simulink library "lib_dGrid"  (R2023b)
settings: Solver=VariableStepAuto  StartTime=0.0  StopTime=10.0  RelTol=1e-3
values from neighbouring files (symbols this model uses):
  C_PM = 10e-3    (= 0.01)    [my_MMC_param.m]
  Cbase = 1/Zbase/wb    (= 3.10849498226e-05)    [my_MMC_param.m]
  f0 = 50/fb    (= 1)    [my_MMC_param.m]
  Fn_filter = 1000    [my_MMC_param.m]
  Fnom = 50    [my_MMC_param.m]
  GFL_APC = 1    [Analysis_Main.m]    (also in initSimu.m; my_MMC_param.m)
  GFL_DVC = 2    [Analysis_Main.m]    (also in initSimu.m; my_MMC_param.m)
  GFM_APC = 3; (values programmed in EMT models)    [Analysis_Main.m]    (also in initSimu.m; my_MMC_param.m = 3)
  GFM_VF = 0    [my_MMC_param.m]
  Ibase = 2*Sbase/(3*Ubase)    [my_MMC_param.m]
  Idcb = Sbase/Udcb    [my_MMC_param.m]
  Ki_Iccsc = 5.15    [my_MMC_param.m]
  Ki_Ireg = CCCTRL.CC.ki    [my_MMC_param.m]
  Ki_Izscc = 100    [my_MMC_param.m]
  Ki_PLL = 1/(CCCTRL.PLL.v0*CCCTRL.PLL.T^2)    [my_MMC_param.m]
  Ki_Preg = 1.0*10    (= 10)    [my_MMC_param.m]
  Ki_Qreg = 1.0*10    (= 10)    [my_MMC_param.m]
  Ki_VAC_GFL = 50    [my_MMC_param.m]
  Ki_VACreg = 10    [my_MMC_param.m]
  Ki_VDCreg = 10    [my_MMC_param.m]
  Ki_WtReg = Kp_WtReg / 0.025    (= 1600)    [my_MMC_param.m]
  Kp_Iccsc = 0.21    [my_MMC_param.m]
  Kp_Ireg = CCCTRL.CC.kp    [my_MMC_param.m]
  Kp_Izscc = 10    [my_MMC_param.m]
  Kp_PLL = 2/CCCTRL.PLL.v0/CCCTRL.PLL.T    [my_MMC_param.m]
  Kp_Preg = 0.5/3*1    (= 0.166666666667)    [my_MMC_param.m]
  Kp_Qreg = 0.5/3*1    (= 0.166666666667)    [my_MMC_param.m]
  Kp_VAC_GFL = 0.5    [my_MMC_param.m]
  Kp_VACreg = 0.01    [my_MMC_param.m]
  Kp_VDCreg = 1    [my_MMC_param.m]
  Kp_WtReg = 40    [my_MMC_param.m]
  Kpv_GFM = 1    [my_MMC_param.m]
  Kpwm = 0.5    [my_MMC_param.m]
  Larm = Larm_pu*(Zbase/wb)    (= 0.0488923985178)    [my_MMC_param.m]
  Lff = Larm_pu/2    (= 0.075)    [my_MMC_param.m]
  Limits_Ireg = [ 2.0  -2.0]    [my_MMC_param.m]
  Limits_Preg = [ 2, -2 ]    [my_MMC_param.m]
  Limits_Qreg = 2*[ 0.42, -0.42 ]    [my_MMC_param.m]
  Limits_VACreg = [ 1.3  -1.3]    [my_MMC_param.m]
  Limits_VDCreg = [ 2.0  -2.0]    [my_MMC_param.m]
  MMC1 = MMC    [Analysis_Main.m]    (also in initSimu.m)
  Nb_PM = 400    [my_MMC_param.m]
  PhaseDelay = 1.0*Ts_Control*2*pi*50    (= 0.0628318530718)    [my_MMC_param.m]
  Pnom = 1000e6    (= 1000000000)    [my_MMC_param.m]
  Rarm = Rarm_pu*Zbase    (= 0.1536)    [my_MMC_param.m]
  Slope_Pref = 0.5    [my_MMC_param.m]
  Slope_Qref = 0.5    [my_MMC_param.m]
  Slope_Vdc_ref = Vnom_dc/2    (= 320000)    [my_MMC_param.m]
  Tdeblock = 1.5    [my_MMC_param.m]
  Ton_CROSSreg = Ton_PQreg+3    (= 7)    [my_MMC_param.m]
  Ton_PQreg = 4    [my_MMC_param.m]
  Ton_VDCreg = 1.5    [my_MMC_param.m]
  Ts = Ts_Control    (= 0.0002)    [my_MMC_param.m]
  Ts_Control = Ts_Power*2    (= 0.0002)    [my_MMC_param.m]
  Ts_Power = 20e-6 * 5    (= 0.0001)    [my_MMC_param.m]
  Ubase = sqrt(2/3)*Vnom_sec    [my_MMC_param.m]
  Udcb = 2*Ubase    [my_MMC_param.m]
  Vc0_PM = 0    [my_MMC_param.m]
  Vnom_dc = 640e3    (= 640000)    [my_MMC_param.m]
  Vnom_sec = 320e3    (= 320000)    [my_MMC_param.m]
  wb = 2*pi*fb    (= 314.159265359)    [my_MMC_param.m]
  Wt_ref_pu = 0.5 * C_PM * (Vnom_dc/Nb_PM)^2 * Nb_PM * 6 / Pnom    (= 0.03072)    [my_MMC_param.m]
undefined symbols (not defined in the file or in its folder): ControlSampleTime, DiscIntNeverNeededParam, MMC, PLL, VSM
libraries: simulink x50, spsCurrentMeasurementLib x20, spsSecondOrderFilterLib x20, spsDiodeLib x12, spsControlledVoltageSourceLib x12, spsSeriesRLCBranchLib x10, spsFirstOrderFilterLib x9, spsVoltageMeasurementLib x8, spsMeanLib x7, FriedrichLibrary x6, $bdroot x6, powerlib_extras x4
(part 2 of 8)

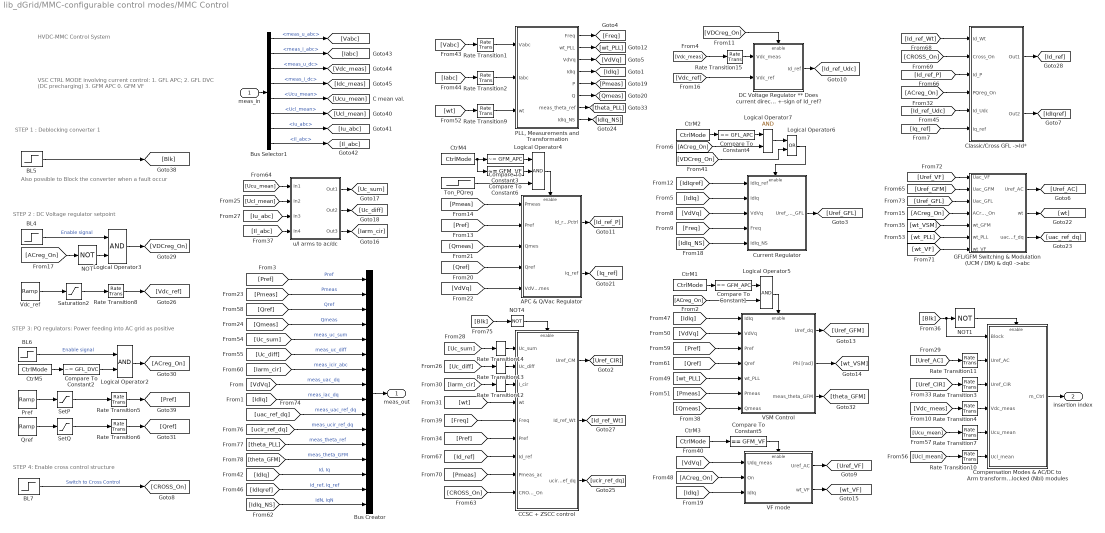
== system lib_dGrid/MMC-configurable control modes/MMC Control ==
  note: HVDC-MMC Control System
  note: VSC CTRL MODE involving current control:
      | 1. GFL APC; 2. GFL DVC  (DC precharging)
      | 3. GFM APC
      | 0. GFM VF
  note: STEP 4: Enable cross control structure
  note: STEP 2 : DC Voltage regulator setpoint
  note: Also possible to Block the converter when a fault occur
  note: STEP 1 : Deblocking converter 1
  note: STEP 3: PQ regulators: Power feeding into
      | AC grid as positive
  meas_in : Inport
  APC & Q/Vac Regulator : Subsystem
  BL4 : Step  Time=Ton_VDCreg  SampleTime=Ts
  BL5 : Step  Time=Tdeblock  Before=1  After=0  SampleTime=Ts_Power
  BL6 : Step  Time=Ton_PQreg  SampleTime=Ts
  BL7 : Step  Time=Ton_CROSSreg  SampleTime=Ts
  Bus Creator : BusCreator  Inputs=16
  Bus Selector1 : BusSelector  OutputSignals=meas_u_abc,meas_i_abc,meas_u_dc,meas_i_dc,Ucu_mean,Ucl_mean,Iu_abc,Il_abc
  CCSC + ZSCC control : Subsystem
  Classic/Cross GFL ->Id* : Subsystem
  Compare To Constant1 : simulink/Logic and Bit Operations/Compare To Constant  relop===  const=GFM_APC  OutDataTypeStr=boolean
  Compare To Constant2 : simulink/Logic and Bit Operations/Compare To Constant  relop=~=  const=GFL_DVC  OutDataTypeStr=boolean
  Compare To Constant3 : simulink/Logic and Bit Operations/Compare To Constant  relop=~=  const=GFM_APC  OutDataTypeStr=boolean
  Compare To Constant4 : simulink/Logic and Bit Operations/Compare To Constant  relop===  const=GFL_APC  OutDataTypeStr=boolean
  Compare To Constant5 : simulink/Logic and Bit Operations/Compare To Constant  relop===  const=GFM_VF  OutDataTypeStr=boolean
  Compare To Constant6 : simulink/Logic and Bit Operations/Compare To Constant  relop=~=  const=GFM_VF  OutDataTypeStr=boolean
  Compensation Modes & AC/DC to Arm transform Number of inserted (Nin) and blocked (Nbl) modules : Subsystem
  CtrM{1..5} (5 alike) : Constant  Value=CtrlMode
  Current Regulator : Subsystem
  DC Voltage Regulator ** Does current direction influence the +-sign of Id_ref? : Subsystem
  GFL/GFM Switching & Modulation (UCM / DM) & dq0 ->abc : Subsystem
  Logical Operator{2..3,5,7} (4 alike) : Logic  AllPortsSameDT=off  OutDataTypeStr=float('double')
  Logical Operator4 : Logic  Inputs=3  AllPortsSameDT=off  OutDataTypeStr=float('double')
  Logical Operator6 : Logic  Operator=OR  AllPortsSameDT=off  OutDataTypeStr=float('double')
  NOT : Logic  Operator=NOT  IconShape=distinctive  AllPortsSameDT=off  OutDataTypeStr=boolean
  NOT1 : Logic  Operator=NOT  IconShape=distinctive  AllPortsSameDT=off  OutDataTypeStr=boolean
  NOT4 : Logic  Operator=NOT  IconShape=distinctive  AllPortsSameDT=off  OutDataTypeStr=boolean
  "PLL, Measurements and Transformation" : Subsystem
  Pref : simulink/Sources/Ramp  slope=Slope_Pref * sign(Set.Pref)  start=Tramping_Pref  InitialOutput=0
  Qref : simulink/Sources/Ramp  slope=Slope_Qref  start=Tramping_Qref  InitialOutput=0
  Rate Transition{1..2,5..6,8..9,12..15} (10 alike) : RateTransition  OutPortSampleTime=Ts_Control
  Rate Transition{3..4,7,10..11} (5 alike) : RateTransition  Deterministic=off  OutPortSampleTime=Ts_Power
  Saturation2 : Saturate  UpperLimit=Vnom_dc  LowerLimit=eps
  SetP : Saturate  UpperLimit=abs(Set.Pref)  LowerLimit=-abs(Set.Pref)
  SetQ : Saturate  UpperLimit=Set.Qref  LowerLimit=-Set.Qref
  Ton_PQreg : Step  Time=Ton_PQreg  SampleTime=Ts
  VF mode : Subsystem
  VSM Control : Subsystem
  "Vdc_ref " : simulink/Sources/Ramp  slope=Slope_Vdc_ref  start=Tramping_Vdc_ref  InitialOutput=Vnom_sec*1.37
  u/l arms to ac/dc : Subsystem
  meas_out : Outport  VectorParamsAs1DForOutWhenUnconnected=off
  insertion index : Outport  Port=2  VectorParamsAs1DForOutWhenUnconnected=off
  wires:
  [Vabc] -> Rate Transition1/1
  [Iabc] -> Rate Transition2/1
  DC Voltage Regulator ** Does current direction influence the +-sign of Id_ref?/1(Id_ref) -> [Id_ref_Udc]
  "PLL, Measurements and Transformation"/2(wt_PLL) -> [wt_PLL]
  "PLL, Measurements and Transformation"/4(IdIq) -> [IdIq]
  [Freq] -> Current Regulator/4(Freq)
  "PLL, Measurements and Transformation"/3(VdVq) -> [VdVq]
  [IdIq] -> Current Regulator/2(IdIq)
  "PLL, Measurements and Transformation"/1(Freq) -> [Freq]
  [VdVq] -> Current Regulator/3(VdVq)
  Rate Transition2/1 -> "PLL, Measurements and Transformation"/2(Iabc)
  Rate Transition1/1 -> "PLL, Measurements and Transformation"/1(Vabc)
  [Vdc_ref] -> DC Voltage Regulator ** Does current direction influence the +-sign of Id_ref?/2(Vdc_ref)
  [VDCreg_On] -> DC Voltage Regulator ** Does current direction influence the +-sign of Id_ref?/Enable
  "PLL, Measurements and Transformation"/5(P) -> [Pmeas]
  [VdVq] -> APC & Q/Vac Regulator/5(VdVq_mes)
  [Qmeas] -> APC & Q/Vac Regulator/3(Qmes)
  "PLL, Measurements and Transformation"/6(Q) -> [Qmeas]
  [Qref] -> APC & Q/Vac Regulator/4(Qref)
  [Uc_diff] -> Rate Transition13/1
  [Iarm_cir] -> Rate Transition12/1
  [Uc_sum] -> Rate Transition14/1
  [Uref_CIR] -> Rate Transition3/1
  Rate Transition11/1 -> Compensation Modes & AC/DC to Arm transform Number of inserted (Nin) and blocked (Nbl) modules/2(Uref_AC)
  Rate Transition3/1 -> Compensation Modes & AC/DC to Arm transform Number of inserted (Nin) and blocked (Nbl) modules/3(Uref_CIR)
  APC & Q/Vac Regulator/1(Id_ref_Pctrl) -> [Id_ref_P]
  [VdVq] -> VSM Control/2(VdVq)
  VSM Control/1(Uref_dq) -> [Uref_GFM]
  [IdIq] -> VSM Control/1(IdIq)
  [Pref] -> VSM Control/3(Pref)
  [wt_PLL] -> VSM Control/5(wt_PLL)
  [wt] -> Rate Transition9/1
  [Freq] -> CCSC + ZSCC control/5(Freq)
  [Pref] -> CCSC + ZSCC control/6(Pref)
  [Vdc_meas] -> Rate Transition4/1
  Rate Transition4/1 -> Compensation Modes & AC/DC to Arm transform Number of inserted (Nin) and blocked (Nbl) modules/4(Vdc_meas)
  CCSC + ZSCC control/2(Id_ref_Wt) -> [Id_ref_Wt]
  [Id_ref] -> CCSC + ZSCC control/7(Id_ref)
  [Pmeas] -> CCSC + ZSCC control/8(Pmeas_ac)
  Rate Transition9/1 -> "PLL, Measurements and Transformation"/3(wt)
  VSM Control/2(Phi [rad]) -> [wt_VSM]
  [wt] -> CCSC + ZSCC control/4(wt)
  [Pmeas] -> VSM Control/6(Pmeas)
  [Qmeas] -> VSM Control/7(Qmeas)
  [Uc_diff] -> Bus Creator/6  "meas_uc_diff"
  [Uc_sum] -> Bus Creator/5  "meas_uc_sum"
  [Iarm_cir] -> Bus Creator/7  "meas_icir_abc"
  Bus Creator/1 -> meas_out/1
  Rate Transition6/1 -> [Qref]
  BL6/1 -> Logical Operator2/1  "Enable signal"
  Pref/1 -> SetP/1
  SetP/1 -> Rate Transition5/1
  BL5/1 -> [Blk]
  BL4/1 -> Logical Operator3/1  "Enable signal"
  Saturation2/1 -> Rate Transition8/1
  BL7/1 -> [CROSS_On]  "Switch to Cross Control"
  "Vdc_ref "/1 -> Saturation2/1
  Rate Transition8/1 -> [Vdc_ref]
  SetQ/1 -> Rate Transition6/1
  Rate Transition5/1 -> [Pref]
  Qref/1 -> SetQ/1
  [CROSS_On] -> CCSC + ZSCC control/9(CROSS_On)
  meas_in/1 -> Bus Selector1/1
  Bus Selector1/7 -> [Iu_abc]  "<Iu_abc>"
  Bus Selector1/8 -> [Il_abc]  "<Il_abc>"
  Bus Selector1/6 -> [Ucl_mean]  "<Ucl_mean>"
  Bus Selector1/5 -> [Ucu_mean]  "<Ucu_mean>"
  Bus Selector1/1 -> [Vabc]  "<meas_u_abc>"
  Bus Selector1/2 -> [Iabc]  "<meas_i_abc>"
  Bus Selector1/3 -> [Vdc_meas]  "<meas_u_dc>"
  Bus Selector1/4 -> [Idc_meas]  "<meas_i_dc>"
  Compensation Modes & AC/DC to Arm transform Number of inserted (Nin) and blocked (Nbl) modules/1(m_Ctrl) -> insertion index/1
  [Ucu_mean] -> Rate Transition7/1
  [Ucl_mean] -> Rate Transition10/1
  Rate Transition7/1 -> Compensation Modes & AC/DC to Arm transform Number of inserted (Nin) and blocked (Nbl) modules/5(Ucu_mean)
  Rate Transition10/1 -> Compensation Modes & AC/DC to Arm transform Number of inserted (Nin) and blocked (Nbl) modules/6(Ucl_mean)
  CCSC + ZSCC control/1(Uref_CM) -> [Uref_CIR]
  [Blk] -> Compensation Modes & AC/DC to Arm transform Number of inserted (Nin) and blocked (Nbl) modules/1(Block), NOT1/1
  [Pref] -> Bus Creator/1  "Pref"
  [Pmeas] -> Bus Creator/2  "Pmeas"
  [Qref] -> Bus Creator/3  "Qref"
  [Qmeas] -> Bus Creator/4  "Qmeas"
  [Pmeas] -> APC & Q/Vac Regulator/1(Pmeas)
  [Pref] -> APC & Q/Vac Regulator/2(Pref)
  APC & Q/Vac Regulator/2(Iq_ref) -> [Iq_ref]
  Compare To Constant2/1 -> Logical Operator2/2
  Logical Operator2/1 -> [ACreg_On]
  [IdIqref] -> Current Regulator/1(IdIq_ref)
  [Id_ref_Wt] -> Classic/Cross GFL ->Id*/1(Id_Wt)
  [CROSS_On] -> Classic/Cross GFL ->Id*/2(Cross_On)
  [Id_ref_P] -> Classic/Cross GFL ->Id*/3(Id_P)
  [ACreg_On] -> Classic/Cross GFL ->Id*/4(PQreg_On)
  [Id_ref_Udc] -> Classic/Cross GFL ->Id*/5(Id_Udc)
  [Iq_ref] -> Classic/Cross GFL ->Id*/6(Iq_ref)
  Classic/Cross GFL ->Id*/1(Out1) -> [Id_ref]
  Classic/Cross GFL ->Id*/2(Out2) -> [IdIqref]
  Logical Operator3/1 -> [VDCreg_On]
  NOT/1 -> Logical Operator3/2
  [ACreg_On] -> NOT/1
  NOT1/1 -> Compensation Modes & AC/DC to Arm transform Number of inserted (Nin) and blocked (Nbl) modules/Enable
  [ACreg_On] -> Logical Operator5/2
  CtrM1/1 -> Compare To Constant1/1
  Compare To Constant1/1 -> Logical Operator5/1
  Logical Operator5/1 -> VSM Control/Enable
  [Qref] -> VSM Control/4(Qref)
  [Uref_AC] -> Rate Transition11/1
  [Uref_GFM] -> GFL/GFM Switching & Modulation (UCM / DM) & dq0 ->abc/2(Uac_GFM)
  [Uref_GFL] -> GFL/GFM Switching & Modulation (UCM / DM) & dq0 ->abc/3(Uac_GFL)
  [ACreg_On] -> GFL/GFM Switching & Modulation (UCM / DM) & dq0 ->abc/4(ACreg_On)
  [wt_VSM] -> GFL/GFM Switching & Modulation (UCM / DM) & dq0 ->abc/5(wt_GFM)
  [wt_PLL] -> GFL/GFM Switching & Modulation (UCM / DM) & dq0 ->abc/6(wt_PLL)
  GFL/GFM Switching & Modulation (UCM / DM) & dq0 ->abc/1(Uref_AC) -> [Uref_AC]
  GFL/GFM Switching & Modulation (UCM / DM) & dq0 ->abc/2(wt) -> [wt]
  [Ucu_mean] -> u/l arms to ac/dc/1(In1)
  [Ucl_mean] -> u/l arms to ac/dc/2(In2)
  [Iu_abc] -> u/l arms to ac/dc/3(In3)
  [Il_abc] -> u/l arms to ac/dc/4(In4)
  u/l arms to ac/dc/1(Out1) -> [Uc_sum]
  u/l arms to ac/dc/2(Out2) -> [Uc_diff]
  u/l arms to ac/dc/3(Out3) -> [Iarm_cir]
  [wt_VF] -> GFL/GFM Switching & Modulation (UCM / DM) & dq0 ->abc/7(wt_VF)
  [Uref_VF] -> GFL/GFM Switching & Modulation (UCM / DM) & dq0 ->abc/1(Uac_VF)
  CCSC + ZSCC control/3(ucir_ref_dq) -> [ucir_ref_dq]
  [ucir_ref_dq] -> Bus Creator/11  "meas_ucir_ref_dq"
  [VdVq] -> Bus Creator/8  "meas_uac_dq"
  [IdIq] -> Bus Creator/9  "meas_iac_dq"
  [uac_ref_dq] -> Bus Creator/10  "meas_uac_ref_dq"
  [theta_PLL] -> Bus Creator/12  "meas_theta_ref"
  [theta_GFM] -> Bus Creator/13  "meas_theta_GFM"
  VSM Control/3(meas_theta_GFM) -> [theta_GFM]
  "PLL, Measurements and Transformation"/7(meas_theta_ref) -> [theta_PLL]
  Current Regulator/1(Uref_AC_GFL) -> [Uref_GFL]
  GFL/GFM Switching & Modulation (UCM / DM) & dq0 ->abc/3(uac_ref_dq) -> [uac_ref_dq]
  [ACreg_On] -> Logical Operator7/2
  [VDCreg_On] -> Logical Operator6/2
  Logical Operator6/1 -> Current Regulator/Enable
  CtrM3/1 -> Compare To Constant5/1
  Compare To Constant5/1 -> VF mode/Enable
  [ACreg_On] -> VF mode/2(On)
  VF mode/2(wt_VF) -> [wt_VF]
  VF mode/1(Uref_AC) -> [Uref_VF]
  [VdVq] -> VF mode/1(Udq_meas)
  [Blk] -> NOT4/1
  NOT4/1 -> CCSC + ZSCC control/Enable
  Ton_PQreg/1 -> Logical Operator4/3
  CtrM2/1 -> Compare To Constant4/1
  Compare To Constant4/1 -> Logical Operator7/1
  Logical Operator7/1 -> Logical Operator6/1
  [IdIq] -> Bus Creator/14  "Id, Iq"
  [IdIqref] -> Bus Creator/15  "Id_ref, Iq_ref"
  Rate Transition12/1 -> CCSC + ZSCC control/3(I_cir)
  Rate Transition13/1 -> CCSC + ZSCC control/2(Uc_diff)
  Rate Transition14/1 -> CCSC + ZSCC control/1(Uc_sum)
  Rate Transition15/1 -> DC Voltage Regulator ** Does current direction influence the +-sign of Id_ref?/1(Vdc_meas)
  [Vdc_meas] -> Rate Transition15/1
  [IdIq] -> VF mode/3(IdIq)
  CtrM5/1 -> Compare To Constant2/1
  CtrM4/1 -> Compare To Constant6/1, Compare To Constant3/1
  Compare To Constant3/1 -> Logical Operator4/1
  Compare To Constant6/1 -> Logical Operator4/2
  Logical Operator4/1 -> APC & Q/Vac Regulator/Enable
  "PLL, Measurements and Transformation"/8(IdIq_NS) -> [IdIq_NS]
  [IdIq_NS] -> Bus Creator/16  "IdN, IqN"
  [IdIq_NS] -> Current Regulator/5(IdIq_NS)

== system lib_dGrid/MMC-configurable control modes/Subsystem ==
  Current Measurement1 : spsCurrentMeasurementLib/Current Measurement  PhasorSimulation=off  OutputType=Complex  PSBequivalent=0
  Goto19 : Goto  Commented=on  GotoTag=V12_Ap
  Voltage Measurement : spsVoltageMeasurementLib/Voltage Measurement  Commented=on  PhasorSimulation=off  OutputType=Complex  PSBequivalent=0
  I1 : PMIOPort  Side=Left
  I2 : PMIOPort  Port=2  Side=Left
  O1 : PMIOPort  Port=3  Side=Right
  O2 : PMIOPort  Port=4  Side=Right
  I_Ap : Outport  VectorParamsAs1DForOutWhenUnconnected=off
  wires:
  Current Measurement1/1 -> I_Ap/1
  Voltage Measurement/1 -> Goto19/1
  connections:
  Current Measurement1/RConn1 -- Voltage Measurement/LConn1 -- I1/RConn1
  Current Measurement1/LConn1 -- O1/RConn1
  I2/RConn1 -- Voltage Measurement/LConn2 -- O2/RConn1

== system lib_dGrid/MMC-configurable control modes/Subsystem1 ==
  Current Measurement1 : spsCurrentMeasurementLib/Current Measurement  PhasorSimulation=off  OutputType=Complex  PSBequivalent=0
  Goto19 : Goto  Commented=on  GotoTag=V12_Am
  Voltage Measurement : spsVoltageMeasurementLib/Voltage Measurement  Commented=on  PhasorSimulation=off  OutputType=Complex  PSBequivalent=0
  I1 : PMIOPort  Side=Left
  I2 : PMIOPort  Port=2  Side=Left
  O1 : PMIOPort  Port=3  Side=Right
  O2 : PMIOPort  Port=4  Side=Right
  I_Am : Outport  VectorParamsAs1DForOutWhenUnconnected=off
  wires:
  Voltage Measurement/1 -> Goto19/1
  Current Measurement1/1 -> I_Am/1
  connections:
  Voltage Measurement/LConn2 -- O2/RConn1 -- I2/RConn1
  Current Measurement1/LConn1 -- O1/RConn1
  Voltage Measurement/LConn1 -- Current Measurement1/RConn1 -- I1/RConn1

== system lib_dGrid/MMC-configurable control modes/Subsystem2 ==
  Current Measurement1 : spsCurrentMeasurementLib/Current Measurement  PhasorSimulation=off  OutputType=Complex  PSBequivalent=0
  Goto19 : Goto  Commented=on  GotoTag=V12_Bp
  Voltage Measurement : spsVoltageMeasurementLib/Voltage Measurement  Commented=on  PhasorSimulation=off  OutputType=Complex  PSBequivalent=0
  I1 : PMIOPort  Side=Left
  I2 : PMIOPort  Port=2  Side=Left
  O1 : PMIOPort  Port=3  Side=Right
  O2 : PMIOPort  Port=4  Side=Right
  I_Bp : Outport  VectorParamsAs1DForOutWhenUnconnected=off
  wires:
  Voltage Measurement/1 -> Goto19/1
  Current Measurement1/1 -> I_Bp/1
  connections:
  Voltage Measurement/LConn2 -- O2/RConn1 -- I2/RConn1
  Current Measurement1/LConn1 -- O1/RConn1
  Voltage Measurement/LConn1 -- Current Measurement1/RConn1 -- I1/RConn1

== system lib_dGrid/MMC-configurable control modes/Subsystem3 ==
  Current Measurement1 : spsCurrentMeasurementLib/Current Measurement  PhasorSimulation=off  OutputType=Complex  PSBequivalent=0
  Goto19 : Goto  Commented=on  GotoTag=V12_Bm
  Voltage Measurement : spsVoltageMeasurementLib/Voltage Measurement  Commented=on  PhasorSimulation=off  OutputType=Complex  PSBequivalent=0
  I1 : PMIOPort  Side=Left
  I2 : PMIOPort  Port=2  Side=Left
  O1 : PMIOPort  Port=3  Side=Right
  O2 : PMIOPort  Port=4  Side=Right
  I_Bm : Outport  VectorParamsAs1DForOutWhenUnconnected=off
  wires:
  Current Measurement1/1 -> I_Bm/1
  Voltage Measurement/1 -> Goto19/1
  connections:
  I1/RConn1 -- Current Measurement1/RConn1 -- Voltage Measurement/LConn1
  Current Measurement1/LConn1 -- O1/RConn1
  I2/RConn1 -- O2/RConn1 -- Voltage Measurement/LConn2

== system lib_dGrid/MMC-configurable control modes/Subsystem4 ==
  Current Measurement1 : spsCurrentMeasurementLib/Current Measurement  PhasorSimulation=off  OutputType=Complex  PSBequivalent=0
  Goto19 : Goto  Commented=on  GotoTag=V12_Cp
  Voltage Measurement : spsVoltageMeasurementLib/Voltage Measurement  Commented=on  PhasorSimulation=off  OutputType=Complex  PSBequivalent=0
  I1 : PMIOPort  Side=Left
  I2 : PMIOPort  Port=2  Side=Left
  O1 : PMIOPort  Port=3  Side=Right
  O2 : PMIOPort  Port=4  Side=Right
  I_Cp : Outport  VectorParamsAs1DForOutWhenUnconnected=off
  wires:
  Current Measurement1/1 -> I_Cp/1
  Voltage Measurement/1 -> Goto19/1
  connections:
  I1/RConn1 -- Current Measurement1/RConn1 -- Voltage Measurement/LConn1
  Current Measurement1/LConn1 -- O1/RConn1
  I2/RConn1 -- O2/RConn1 -- Voltage Measurement/LConn2

== system lib_dGrid/MMC-configurable control modes/Subsystem5 ==
  Current Measurement1 : spsCurrentMeasurementLib/Current Measurement  PhasorSimulation=off  OutputType=Complex  PSBequivalent=0
  Goto19 : Goto  Commented=on  GotoTag=V12_Cm
  Voltage Measurement : spsVoltageMeasurementLib/Voltage Measurement  Commented=on  PhasorSimulation=off  OutputType=Complex  PSBequivalent=0
  I1 : PMIOPort  Side=Left
  I2 : PMIOPort  Port=2  Side=Left
  O1 : PMIOPort  Port=3  Side=Right
  O2 : PMIOPort  Port=4  Side=Right
  I_Cm : Outport  VectorParamsAs1DForOutWhenUnconnected=off
  wires:
  Voltage Measurement/1 -> Goto19/1
  Current Measurement1/1 -> I_Cm/1
  connections:
  Voltage Measurement/LConn2 -- O2/RConn1 -- I2/RConn1
  Current Measurement1/LConn1 -- O1/RConn1
  Voltage Measurement/LConn1 -- Current Measurement1/RConn1 -- I1/RConn1

== system lib_dGrid/TL-VSC-configurable control modes/Filters 60Hz2 ==
  note: High-pass
      | damped filters
  note: AC Filters, 40 Mvar @ 100 kV
  "27th 18 Mvar Q = 15 " : spsThreePhaseHarmonicFilterLib/Three-Phase Harmonic Filter  LConnTagsString=A|B|C  FilterType=High-pass  FilterConnection=Y (grounded)  ParNom="[320e3  Fnom]"  Qc=0.2*Pnom * 0.45  Fr=27*Fnom  Frd=[11*60 13*60]  Q=15  Measurements=None
      settings: AttributesFormatString=\n
  "54th 22 Mvar Q = 15 " : spsThreePhaseHarmonicFilterLib/Three-Phase Harmonic Filter  LConnTagsString=A|B|C  FilterType=High-pass  FilterConnection=Y (grounded)  ParNom="[320e3  Fnom]"  Qc=0.2*Pnom * 0.55  Fr=(2*27)*Fnom  Frd=[11*60 13*60]  Q=15  Measurements=None
      settings: AttributesFormatString=\n
  A : PMIOPort  Side=Left
  B : PMIOPort  Port=2  Side=Left
  C : PMIOPort  Port=3  Side=Left
  connections:
  "54th 22 Mvar Q = 15 "/LConn3 -- C/RConn1 -- "27th 18 Mvar Q = 15 "/LConn3
  "54th 22 Mvar Q = 15 "/LConn2 -- B/RConn1 -- "27th 18 Mvar Q = 15 "/LConn2
  "54th 22 Mvar Q = 15 "/LConn1 -- A/RConn1 -- "27th 18 Mvar Q = 15 "/LConn1

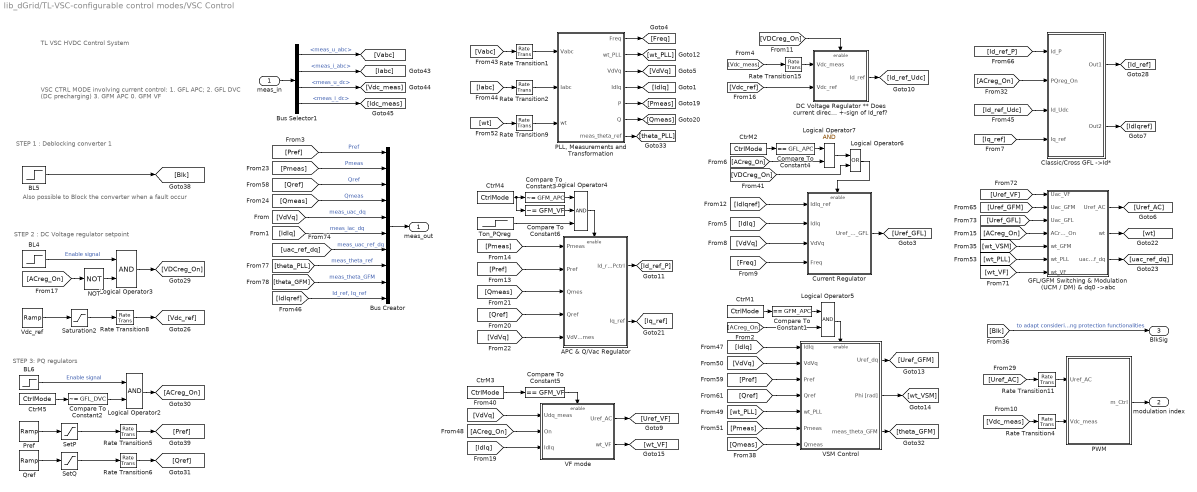
== system lib_dGrid/TL-VSC-configurable control modes/VSC Control ==
  note: TL VSC HVDC
      | Control System
  note: VSC CTRL MODE involving current control:
      | 1. GFL APC; 2. GFL DVC  (DC precharging)
      | 3. GFM APC
      | 0. GFM VF
  note: STEP 2 : DC Voltage regulator setpoint
  note: Also possible to Block the converter when a fault occur
  note: STEP 1 : Deblocking converter 1
  note: STEP 3: PQ regulators
  meas_in : Inport
  APC & Q/Vac Regulator : Subsystem
  BL4 : Step  Time=Ton_VDCreg  SampleTime=Ts
  BL5 : Step  Time=Tdeblock  Before=1  After=0  SampleTime=Ts_Power
  BL6 : Step  Time=Ton_PQreg  SampleTime=Ts
  Bus Creator : BusCreator  Inputs=10
  Bus Selector1 : BusSelector  OutputSignals=meas_u_abc,meas_i_abc,meas_u_dc,meas_i_dc
  Classic/Cross GFL ->Id* : Subsystem
  Compare To Constant1 : simulink/Logic and Bit Operations/Compare To Constant  relop===  const=GFM_APC  OutDataTypeStr=boolean
  Compare To Constant2 : simulink/Logic and Bit Operations/Compare To Constant  relop=~=  const=GFL_DVC  OutDataTypeStr=boolean
  Compare To Constant3 : simulink/Logic and Bit Operations/Compare To Constant  relop=~=  const=GFM_APC  OutDataTypeStr=boolean
  Compare To Constant4 : simulink/Logic and Bit Operations/Compare To Constant  relop===  const=GFL_APC  OutDataTypeStr=boolean
  Compare To Constant5 : simulink/Logic and Bit Operations/Compare To Constant  relop===  const=GFM_VF  OutDataTypeStr=boolean
  Compare To Constant6 : simulink/Logic and Bit Operations/Compare To Constant  relop=~=  const=GFM_VF  OutDataTypeStr=boolean
  CtrM{1..5} (5 alike) : Constant  Value=CtrlMode
  Current Regulator : Subsystem
  DC Voltage Regulator ** Does current direction influence the +-sign of Id_ref? : Subsystem
  GFL/GFM Switching & Modulation (UCM / DM) & dq0 ->abc : Subsystem
  Logical Operator{2..3,5,7} (4 alike) : Logic  AllPortsSameDT=off  OutDataTypeStr=float('double')
  Logical Operator4 : Logic  Inputs=3  AllPortsSameDT=off  OutDataTypeStr=float('double')
  Logical Operator6 : Logic  Operator=OR  AllPortsSameDT=off  OutDataTypeStr=float('double')
  NOT : Logic  Operator=NOT  IconShape=distinctive  AllPortsSameDT=off  OutDataTypeStr=boolean
  "PLL, Measurements and Transformation" : Subsystem
  PWM : Subsystem
  Pref : simulink/Sources/Ramp  slope=Slope_Pref  start=Tramping_Pref  InitialOutput=0
  Qref : simulink/Sources/Ramp  slope=Slope_Qref  start=Tramping_Qref  InitialOutput=0
  Rate Transition{1..2,5..6,8..9,15} (7 alike) : RateTransition  OutPortSampleTime=Ts_Control
  Rate Transition11 : RateTransition  Deterministic=off  OutPortSampleTime=Ts_Power
  Rate Transition4 : RateTransition  Deterministic=off  OutPortSampleTime=Ts_Power
  Saturation2 : Saturate  UpperLimit=Vnom_dc  LowerLimit=eps
  SetP : Saturate  UpperLimit=Set.Pref  LowerLimit=-Set.Pref
  SetQ : Saturate  UpperLimit=Set.Qref  LowerLimit=-Set.Qref
  Ton_PQreg : Step  Time=Ton_PQreg  SampleTime=Ts
  VF mode : Subsystem
  VSM Control : Subsystem
  "Vdc_ref " : simulink/Sources/Ramp  slope=Slope_Vdc_ref  start=Tramping_Vdc_ref  InitialOutput=Vnom_sec*1.37
  meas_out : Outport  VectorParamsAs1DForOutWhenUnconnected=off
  modulation index : Outport  Port=2  VectorParamsAs1DForOutWhenUnconnected=off
  BlkSig : Outport  Port=3  VectorParamsAs1DForOutWhenUnconnected=off
  wires:
  [Vabc] -> Rate Transition1/1
  [Iabc] -> Rate Transition2/1
  DC Voltage Regulator ** Does current direction influence the +-sign of Id_ref?/1(Id_ref) -> [Id_ref_Udc]
  "PLL, Measurements and Transformation"/2(wt_PLL) -> [wt_PLL]
  "PLL, Measurements and Transformation"/4(IdIq) -> [IdIq]
  [Freq] -> Current Regulator/4(Freq)
  "PLL, Measurements and Transformation"/3(VdVq) -> [VdVq]
  [IdIq] -> Current Regulator/2(IdIq)
  "PLL, Measurements and Transformation"/1(Freq) -> [Freq]
  [VdVq] -> Current Regulator/3(VdVq)
  Rate Transition2/1 -> "PLL, Measurements and Transformation"/2(Iabc)
  Rate Transition1/1 -> "PLL, Measurements and Transformation"/1(Vabc)
  [Vdc_ref] -> DC Voltage Regulator ** Does current direction influence the +-sign of Id_ref?/2(Vdc_ref)
  [VDCreg_On] -> DC Voltage Regulator ** Does current direction influence the +-sign of Id_ref?/Enable
  "PLL, Measurements and Transformation"/5(P) -> [Pmeas]
  [VdVq] -> APC & Q/Vac Regulator/5(VdVq_mes)
  [Qmeas] -> APC & Q/Vac Regulator/3(Qmes)
  "PLL, Measurements and Transformation"/6(Q) -> [Qmeas]
  [Qref] -> APC & Q/Vac Regulator/4(Qref)
  Rate Transition11/1 -> PWM/1(Uref_AC)
  APC & Q/Vac Regulator/1(Id_ref_Pctrl) -> [Id_ref_P]
  [VdVq] -> VSM Control/2(VdVq)
  VSM Control/1(Uref_dq) -> [Uref_GFM]
  [IdIq] -> VSM Control/1(IdIq)
  [Pref] -> VSM Control/3(Pref)
  [wt_PLL] -> VSM Control/5(wt_PLL)
  [wt] -> Rate Transition9/1
  [Vdc_meas] -> Rate Transition4/1
  Rate Transition4/1 -> PWM/2(Vdc_meas)
  Rate Transition9/1 -> "PLL, Measurements and Transformation"/3(wt)
  VSM Control/2(Phi [rad]) -> [wt_VSM]
  [Pmeas] -> VSM Control/6(Pmeas)
  [Qmeas] -> VSM Control/7(Qmeas)
  Bus Creator/1 -> meas_out/1
  Rate Transition6/1 -> [Qref]
  BL6/1 -> Logical Operator2/1  "Enable signal"
  Pref/1 -> SetP/1
  SetP/1 -> Rate Transition5/1
  BL5/1 -> [Blk]
  BL4/1 -> Logical Operator3/1  "Enable signal"
  Saturation2/1 -> Rate Transition8/1
  "Vdc_ref "/1 -> Saturation2/1
  Rate Transition8/1 -> [Vdc_ref]
  SetQ/1 -> Rate Transition6/1
  Rate Transition5/1 -> [Pref]
  Qref/1 -> SetQ/1
  meas_in/1 -> Bus Selector1/1
  Bus Selector1/1 -> [Vabc]  "<meas_u_abc>"
  Bus Selector1/2 -> [Iabc]  "<meas_i_abc>"
  Bus Selector1/3 -> [Vdc_meas]  "<meas_u_dc>"
  Bus Selector1/4 -> [Idc_meas]  "<meas_i_dc>"
  PWM/1(m_Ctrl) -> modulation index/1
  [Pref] -> Bus Creator/1  "Pref"
  [Pmeas] -> Bus Creator/2  "Pmeas"
  [Qref] -> Bus Creator/3  "Qref"
  [Qmeas] -> Bus Creator/4  "Qmeas"
  [Pmeas] -> APC & Q/Vac Regulator/1(Pmeas)
  [Pref] -> APC & Q/Vac Regulator/2(Pref)
  APC & Q/Vac Regulator/2(Iq_ref) -> [Iq_ref]
  Compare To Constant2/1 -> Logical Operator2/2
  Logical Operator2/1 -> [ACreg_On]
  [IdIqref] -> Current Regulator/1(IdIq_ref)
  [Id_ref_P] -> Classic/Cross GFL ->Id*/1(Id_P)
  [ACreg_On] -> Classic/Cross GFL ->Id*/2(PQreg_On)
  [Id_ref_Udc] -> Classic/Cross GFL ->Id*/3(Id_Udc)
  [Iq_ref] -> Classic/Cross GFL ->Id*/4(Iq_ref)
  Classic/Cross GFL ->Id*/1(Out1) -> [Id_ref]
  Classic/Cross GFL ->Id*/2(Out2) -> [IdIqref]
  Logical Operator3/1 -> [VDCreg_On]
  NOT/1 -> Logical Operator3/2
  [ACreg_On] -> NOT/1
  [ACreg_On] -> Logical Operator5/2
  CtrM1/1 -> Compare To Constant1/1
  Compare To Constant1/1 -> Logical Operator5/1
  Logical Operator5/1 -> VSM Control/Enable
  [Qref] -> VSM Control/4(Qref)
  [Uref_AC] -> Rate Transition11/1
  [Uref_GFM] -> GFL/GFM Switching & Modulation (UCM / DM) & dq0 ->abc/2(Uac_GFM)
  [Uref_GFL] -> GFL/GFM Switching & Modulation (UCM / DM) & dq0 ->abc/3(Uac_GFL)
  [ACreg_On] -> GFL/GFM Switching & Modulation (UCM / DM) & dq0 ->abc/4(ACreg_On)
  [wt_VSM] -> GFL/GFM Switching & Modulation (UCM / DM) & dq0 ->abc/5(wt_GFM)
  [wt_PLL] -> GFL/GFM Switching & Modulation (UCM / DM) & dq0 ->abc/6(wt_PLL)
  GFL/GFM Switching & Modulation (UCM / DM) & dq0 ->abc/1(Uref_AC) -> [Uref_AC]
  GFL/GFM Switching & Modulation (UCM / DM) & dq0 ->abc/2(wt) -> [wt]
  [wt_VF] -> GFL/GFM Switching & Modulation (UCM / DM) & dq0 ->abc/7(wt_VF)
  [Uref_VF] -> GFL/GFM Switching & Modulation (UCM / DM) & dq0 ->abc/1(Uac_VF)
  VSM Control/3(meas_theta_GFM) -> [theta_GFM]
  "PLL, Measurements and Transformation"/7(meas_theta_ref) -> [theta_PLL]
  Current Regulator/1(Uref_AC_GFL) -> [Uref_GFL]
  GFL/GFM Switching & Modulation (UCM / DM) & dq0 ->abc/3(uac_ref_dq) -> [uac_ref_dq]
  [ACreg_On] -> Logical Operator7/2
  [VDCreg_On] -> Logical Operator6/2
  Logical Operator6/1 -> Current Regulator/Enable
  CtrM3/1 -> Compare To Constant5/1
  Compare To Constant5/1 -> VF mode/Enable
  [ACreg_On] -> VF mode/2(On)
  VF mode/2(wt_VF) -> [wt_VF]
  VF mode/1(Uref_AC) -> [Uref_VF]
  [VdVq] -> VF mode/1(Udq_meas)
  Ton_PQreg/1 -> Logical Operator4/3
  CtrM2/1 -> Compare To Constant4/1
  Compare To Constant4/1 -> Logical Operator7/1
  Logical Operator7/1 -> Logical Operator6/1
  Rate Transition15/1 -> DC Voltage Regulator ** Does current direction influence the +-sign of Id_ref?/1(Vdc_meas)
  [Vdc_meas] -> Rate Transition15/1
  [IdIq] -> VF mode/3(IdIq)
  CtrM5/1 -> Compare To Constant2/1
  CtrM4/1 -> Compare To Constant6/1, Compare To Constant3/1
  Compare To Constant3/1 -> Logical Operator4/1
  Compare To Constant6/1 -> Logical Operator4/2
  Logical Operator4/1 -> APC & Q/Vac Regulator/Enable
  [IdIq] -> Bus Creator/6  "meas_iac_dq"
  [uac_ref_dq] -> Bus Creator/7  "meas_uac_ref_dq"
  [VdVq] -> Bus Creator/5  "meas_uac_dq"
  [theta_GFM] -> Bus Creator/9  "meas_theta_GFM"
  [theta_PLL] -> Bus Creator/8  "meas_theta_ref"
  [IdIqref] -> Bus Creator/10  "Id_ref, Iq_ref"
  [Blk] -> BlkSig/1  "to adapt considering protection functionalities"

== system lib_dGrid/MMC-configurable control modes/Half-Bridge MMC Am/HalfBridgeMMC_Agt_Discrete ==
  N : Inport  PortDimensions=2
  Current Measurement1 : spsCurrentMeasurementLib/Current Measurement  PhasorSimulation=off  OutputType=Complex  PSBequivalent=0
  Current Measurement2 : spsCurrentMeasurementLib/Current Measurement  PhasorSimulation=off  OutputType=Complex  PSBequivalent=0
  Demux : Demux  Outputs=2
  Discrete-Time Integrator : DiscreteIntegrator  IntegratorMethod=Integration: Trapezoidal  gainval=1  InitialCondition=Vc_Initial  SampleTime=Ts  UpperSaturationLimit=5000  LowerSaturationLimit=500  ICPrevOutput=DiscIntNeverNeededParam  ICPrevScaledInput=DiscIntNeverNeededParam
  Dp : spsDiodeLib/Diode  Ron=Ron_Diode  Lon=0  Vf=Vf_Diode  IC=0  UseSnubber=off  Rs=Rs_Diode  Cs=Cs_Diode  Measurements=off
  Dp2 : spsDiodeLib/Diode  Ron=Ron_Diode  Lon=0  Vf=Vf_Diode  IC=0  UseSnubber=off  Rs=Rs_Diode  Cs=Cs_Diode  Measurements=off
  Gain : Gain  Gain=1/(C*n)
  Gain2 : Gain  Gain=2
  Mux : Mux  Inputs=2
  Product1 : Product
  Product2 : Product
  Saturation1 : Saturate  UpperLimit=n  LowerLimit=0
  Sum1 : Sum  Inputs=1  InputSameDT=on  SaturateOnIntegerOverflow=on  OutDataTypeStr=Inherit: Same as first input
  Sum2 : Sum  Inputs=+-  InputSameDT=on  SaturateOnIntegerOverflow=on  OutDataTypeStr=Inherit: Same as first input
  Unit Delay1 : UnitDelay  SampleTime=Ts  HasFrameUpgradeWarning=on
  Unit Delay3 : UnitDelay  InitialCondition=Vc_Initial  SampleTime=Ts  HasFrameUpgradeWarning=on
  Unit Delay4 : UnitDelay  InitialCondition=Vc_Initial  SampleTime=Ts  HasFrameUpgradeWarning=on
  Vp : spsControlledVoltageSourceLib/Controlled Voltage Source  Initialize=off  Source_Type=AC  Amplitude=0  Phase=0  Frequency=0  Measurements=None
  Vp1 : spsControlledVoltageSourceLib/Controlled Voltage Source  Initialize=off  Source_Type=AC  Amplitude=0  Phase=0  Frequency=0  Measurements=None
  1 : PMIOPort  Side=Left
  2 : PMIOPort  Port=2  Side=Left
  Vc : Outport  VectorParamsAs1DForOutWhenUnconnected=off
  wires:
  N/1 -> Saturation1/1
  [Imod] -> Mux/1
  Unit Delay3/1 -> Sum2/2
  Unit Delay4/1 -> Unit Delay3/1, Gain2/1
  Gain2/1 -> Sum2/1
  Gain/1 -> Discrete-Time Integrator/1
  Discrete-Time Integrator/1 -> Unit Delay4/1
  Mux/1 -> Unit Delay1/1
  Product2/1 -> Demux/1
  Demux/1 -> [Vin]
  Demux/2 -> [Vbl]
  [Vin] -> Vp/1
  Current Measurement1/1 -> [Imod]
  Current Measurement2/1 -> [Icap]
  [Vbl] -> Vp1/1
  [Icap] -> Mux/2
  Unit Delay1/1 -> Product1/2
  Saturation1/1 -> Product1/1, Product2/1
  Product1/1 -> Sum1/1
  Sum2/1 -> Product2/2, Vc/1
  Sum1/1 -> Gain/1
  connections:
  1/RConn1 -- Vp/RConn1
  Vp/LConn1 -- Current Measurement1/LConn1
  Current Measurement1/RConn1 -- Dp/LConn1 -- Dp2/RConn1
  Current Measurement2/LConn1 -- Dp/RConn1
  Vp1/RConn1 -- Current Measurement2/RConn1
  Vp1/LConn1 -- 2/RConn1 -- Dp2/LConn1

== system lib_dGrid/MMC-configurable control modes/Half-Bridge MMC Ap/HalfBridgeMMC_Agt_Discrete ==
  N : Inport  PortDimensions=2
  Current Measurement1 : spsCurrentMeasurementLib/Current Measurement  PhasorSimulation=off  OutputType=Complex  PSBequivalent=0
  Current Measurement2 : spsCurrentMeasurementLib/Current Measurement  PhasorSimulation=off  OutputType=Complex  PSBequivalent=0
  Demux : Demux  Outputs=2
  Discrete-Time Integrator : DiscreteIntegrator  IntegratorMethod=Integration: Trapezoidal  gainval=1  InitialCondition=Vc_Initial  SampleTime=Ts  UpperSaturationLimit=5000  LowerSaturationLimit=500  ICPrevOutput=DiscIntNeverNeededParam  ICPrevScaledInput=DiscIntNeverNeededParam
  Dp : spsDiodeLib/Diode  Ron=Ron_Diode  Lon=0  Vf=Vf_Diode  IC=0  UseSnubber=off  Rs=Rs_Diode  Cs=Cs_Diode  Measurements=off
  Dp2 : spsDiodeLib/Diode  Ron=Ron_Diode  Lon=0  Vf=Vf_Diode  IC=0  UseSnubber=off  Rs=Rs_Diode  Cs=Cs_Diode  Measurements=off
  Gain : Gain  Gain=1/(C*n)
  Gain2 : Gain  Gain=2
  Mux : Mux  Inputs=2
  Product1 : Product
  Product2 : Product
  Saturation1 : Saturate  UpperLimit=n  LowerLimit=0
  Sum1 : Sum  Inputs=1  InputSameDT=on  SaturateOnIntegerOverflow=on  OutDataTypeStr=Inherit: Same as first input
  Sum2 : Sum  Inputs=+-  InputSameDT=on  SaturateOnIntegerOverflow=on  OutDataTypeStr=Inherit: Same as first input
  Unit Delay1 : UnitDelay  SampleTime=Ts  HasFrameUpgradeWarning=on
  Unit Delay3 : UnitDelay  InitialCondition=Vc_Initial  SampleTime=Ts  HasFrameUpgradeWarning=on
  Unit Delay4 : UnitDelay  InitialCondition=Vc_Initial  SampleTime=Ts  HasFrameUpgradeWarning=on
  Vp : spsControlledVoltageSourceLib/Controlled Voltage Source  Initialize=off  Source_Type=AC  Amplitude=0  Phase=0  Frequency=0  Measurements=None
  Vp1 : spsControlledVoltageSourceLib/Controlled Voltage Source  Initialize=off  Source_Type=AC  Amplitude=0  Phase=0  Frequency=0  Measurements=None
  1 : PMIOPort  Side=Left
  2 : PMIOPort  Port=2  Side=Left
  Vc : Outport  VectorParamsAs1DForOutWhenUnconnected=off
  wires:
  Sum1/1 -> Gain/1
  Sum2/1 -> Vc/1, Product2/2
  Product1/1 -> Sum1/1
  Saturation1/1 -> Product2/1, Product1/1
  Unit Delay1/1 -> Product1/2
  [Icap] -> Mux/2
  [Vbl] -> Vp1/1
  Current Measurement2/1 -> [Icap]
  Current Measurement1/1 -> [Imod]
  [Vin] -> Vp/1
  Demux/2 -> [Vbl]
  Demux/1 -> [Vin]
  Product2/1 -> Demux/1
  Mux/1 -> Unit Delay1/1
  Discrete-Time Integrator/1 -> Unit Delay4/1
  Gain/1 -> Discrete-Time Integrator/1
  Gain2/1 -> Sum2/1
  Unit Delay4/1 -> Gain2/1, Unit Delay3/1
  Unit Delay3/1 -> Sum2/2
  [Imod] -> Mux/1
  N/1 -> Saturation1/1
  connections:
  Dp2/LConn1 -- 2/RConn1 -- Vp1/LConn1
  Vp1/RConn1 -- Current Measurement2/RConn1
  Current Measurement2/LConn1 -- Dp/RConn1
  Dp2/RConn1 -- Dp/LConn1 -- Current Measurement1/RConn1
  Vp/LConn1 -- Current Measurement1/LConn1
  1/RConn1 -- Vp/RConn1

== system lib_dGrid/MMC-configurable control modes/Half-Bridge MMC Bm/HalfBridgeMMC_Agt_Discrete ==
  N : Inport  PortDimensions=2
  Current Measurement1 : spsCurrentMeasurementLib/Current Measurement  PhasorSimulation=off  OutputType=Complex  PSBequivalent=0
  Current Measurement2 : spsCurrentMeasurementLib/Current Measurement  PhasorSimulation=off  OutputType=Complex  PSBequivalent=0
  Demux : Demux  Outputs=2
  Discrete-Time Integrator : DiscreteIntegrator  IntegratorMethod=Integration: Trapezoidal  gainval=1  InitialCondition=Vc_Initial  SampleTime=Ts  UpperSaturationLimit=5000  LowerSaturationLimit=500  ICPrevOutput=DiscIntNeverNeededParam  ICPrevScaledInput=DiscIntNeverNeededParam
  Dp : spsDiodeLib/Diode  Ron=Ron_Diode  Lon=0  Vf=Vf_Diode  IC=0  UseSnubber=off  Rs=Rs_Diode  Cs=Cs_Diode  Measurements=off
  Dp2 : spsDiodeLib/Diode  Ron=Ron_Diode  Lon=0  Vf=Vf_Diode  IC=0  UseSnubber=off  Rs=Rs_Diode  Cs=Cs_Diode  Measurements=off
  Gain : Gain  Gain=1/(C*n)
  Gain2 : Gain  Gain=2
  Mux : Mux  Inputs=2
  Product1 : Product
  Product2 : Product
  Saturation1 : Saturate  UpperLimit=n  LowerLimit=0
  Sum1 : Sum  Inputs=1  InputSameDT=on  SaturateOnIntegerOverflow=on  OutDataTypeStr=Inherit: Same as first input
  Sum2 : Sum  Inputs=+-  InputSameDT=on  SaturateOnIntegerOverflow=on  OutDataTypeStr=Inherit: Same as first input
  Unit Delay1 : UnitDelay  SampleTime=Ts  HasFrameUpgradeWarning=on
  Unit Delay3 : UnitDelay  InitialCondition=Vc_Initial  SampleTime=Ts  HasFrameUpgradeWarning=on
  Unit Delay4 : UnitDelay  InitialCondition=Vc_Initial  SampleTime=Ts  HasFrameUpgradeWarning=on
  Vp : spsControlledVoltageSourceLib/Controlled Voltage Source  Initialize=off  Source_Type=AC  Amplitude=0  Phase=0  Frequency=0  Measurements=None
  Vp1 : spsControlledVoltageSourceLib/Controlled Voltage Source  Initialize=off  Source_Type=AC  Amplitude=0  Phase=0  Frequency=0  Measurements=None
  1 : PMIOPort  Side=Left
  2 : PMIOPort  Port=2  Side=Left
  Vc : Outport  VectorParamsAs1DForOutWhenUnconnected=off
  wires:
  Sum1/1 -> Gain/1
  Sum2/1 -> Vc/1, Product2/2
  Product1/1 -> Sum1/1
  Saturation1/1 -> Product2/1, Product1/1
  Unit Delay1/1 -> Product1/2
  [Icap] -> Mux/2
  [Vbl] -> Vp1/1
  Current Measurement2/1 -> [Icap]
  Current Measurement1/1 -> [Imod]
  [Vin] -> Vp/1
  Demux/2 -> [Vbl]
  Demux/1 -> [Vin]
  Product2/1 -> Demux/1
  Mux/1 -> Unit Delay1/1
  Discrete-Time Integrator/1 -> Unit Delay4/1
  Gain/1 -> Discrete-Time Integrator/1
  Gain2/1 -> Sum2/1
  Unit Delay4/1 -> Gain2/1, Unit Delay3/1
  Unit Delay3/1 -> Sum2/2
  [Imod] -> Mux/1
  N/1 -> Saturation1/1
  connections:
  Dp2/LConn1 -- 2/RConn1 -- Vp1/LConn1
  Vp1/RConn1 -- Current Measurement2/RConn1
  Current Measurement2/LConn1 -- Dp/RConn1
  Dp2/RConn1 -- Dp/LConn1 -- Current Measurement1/RConn1
  Vp/LConn1 -- Current Measurement1/LConn1
  1/RConn1 -- Vp/RConn1

== system lib_dGrid/MMC-configurable control modes/Half-Bridge MMC Bp/HalfBridgeMMC_Agt_Discrete ==
  N : Inport  PortDimensions=2
  Current Measurement1 : spsCurrentMeasurementLib/Current Measurement  PhasorSimulation=off  OutputType=Complex  PSBequivalent=0
  Current Measurement2 : spsCurrentMeasurementLib/Current Measurement  PhasorSimulation=off  OutputType=Complex  PSBequivalent=0
  Demux : Demux  Outputs=2
  Discrete-Time Integrator : DiscreteIntegrator  IntegratorMethod=Integration: Trapezoidal  gainval=1  InitialCondition=Vc_Initial  SampleTime=Ts  UpperSaturationLimit=5000  LowerSaturationLimit=500  ICPrevOutput=DiscIntNeverNeededParam  ICPrevScaledInput=DiscIntNeverNeededParam
  Dp : spsDiodeLib/Diode  Ron=Ron_Diode  Lon=0  Vf=Vf_Diode  IC=0  UseSnubber=off  Rs=Rs_Diode  Cs=Cs_Diode  Measurements=off
  Dp2 : spsDiodeLib/Diode  Ron=Ron_Diode  Lon=0  Vf=Vf_Diode  IC=0  UseSnubber=off  Rs=Rs_Diode  Cs=Cs_Diode  Measurements=off
  Gain : Gain  Gain=1/(C*n)
  Gain2 : Gain  Gain=2
  Mux : Mux  Inputs=2
  Product1 : Product
  Product2 : Product
  Saturation1 : Saturate  UpperLimit=n  LowerLimit=0
  Sum1 : Sum  Inputs=1  InputSameDT=on  SaturateOnIntegerOverflow=on  OutDataTypeStr=Inherit: Same as first input
  Sum2 : Sum  Inputs=+-  InputSameDT=on  SaturateOnIntegerOverflow=on  OutDataTypeStr=Inherit: Same as first input
  Unit Delay1 : UnitDelay  SampleTime=Ts  HasFrameUpgradeWarning=on
  Unit Delay3 : UnitDelay  InitialCondition=Vc_Initial  SampleTime=Ts  HasFrameUpgradeWarning=on
  Unit Delay4 : UnitDelay  InitialCondition=Vc_Initial  SampleTime=Ts  HasFrameUpgradeWarning=on
  Vp : spsControlledVoltageSourceLib/Controlled Voltage Source  Initialize=off  Source_Type=AC  Amplitude=0  Phase=0  Frequency=0  Measurements=None
  Vp1 : spsControlledVoltageSourceLib/Controlled Voltage Source  Initialize=off  Source_Type=AC  Amplitude=0  Phase=0  Frequency=0  Measurements=None
  1 : PMIOPort  Side=Left
  2 : PMIOPort  Port=2  Side=Left
  Vc : Outport  VectorParamsAs1DForOutWhenUnconnected=off
  wires:
  N/1 -> Saturation1/1
  [Imod] -> Mux/1
  Unit Delay3/1 -> Sum2/2
  Unit Delay4/1 -> Unit Delay3/1, Gain2/1
  Gain2/1 -> Sum2/1
  Gain/1 -> Discrete-Time Integrator/1
  Discrete-Time Integrator/1 -> Unit Delay4/1
  Mux/1 -> Unit Delay1/1
  Product2/1 -> Demux/1
  Demux/1 -> [Vin]
  Demux/2 -> [Vbl]
  [Vin] -> Vp/1
  Current Measurement1/1 -> [Imod]
  Current Measurement2/1 -> [Icap]
  [Vbl] -> Vp1/1
  [Icap] -> Mux/2
  Unit Delay1/1 -> Product1/2
  Saturation1/1 -> Product1/1, Product2/1
  Product1/1 -> Sum1/1
  Sum2/1 -> Product2/2, Vc/1
  Sum1/1 -> Gain/1
  connections:
  1/RConn1 -- Vp/RConn1
  Vp/LConn1 -- Current Measurement1/LConn1
  Current Measurement1/RConn1 -- Dp/LConn1 -- Dp2/RConn1
  Current Measurement2/LConn1 -- Dp/RConn1
  Vp1/RConn1 -- Current Measurement2/RConn1
  Vp1/LConn1 -- 2/RConn1 -- Dp2/LConn1

== system lib_dGrid/MMC-configurable control modes/Half-Bridge MMC Cm/HalfBridgeMMC_Agt_Discrete ==
  N : Inport  PortDimensions=2
  Current Measurement1 : spsCurrentMeasurementLib/Current Measurement  PhasorSimulation=off  OutputType=Complex  PSBequivalent=0
  Current Measurement2 : spsCurrentMeasurementLib/Current Measurement  PhasorSimulation=off  OutputType=Complex  PSBequivalent=0
  Demux : Demux  Outputs=2
  Discrete-Time Integrator : DiscreteIntegrator  IntegratorMethod=Integration: Trapezoidal  gainval=1  InitialCondition=Vc_Initial  SampleTime=Ts  UpperSaturationLimit=5000  LowerSaturationLimit=500  ICPrevOutput=DiscIntNeverNeededParam  ICPrevScaledInput=DiscIntNeverNeededParam
  Dp : spsDiodeLib/Diode  Ron=Ron_Diode  Lon=0  Vf=Vf_Diode  IC=0  UseSnubber=off  Rs=Rs_Diode  Cs=Cs_Diode  Measurements=off
  Dp2 : spsDiodeLib/Diode  Ron=Ron_Diode  Lon=0  Vf=Vf_Diode  IC=0  UseSnubber=off  Rs=Rs_Diode  Cs=Cs_Diode  Measurements=off
  Gain : Gain  Gain=1/(C*n)
  Gain2 : Gain  Gain=2
  Mux : Mux  Inputs=2
  Product1 : Product
  Product2 : Product
  Saturation1 : Saturate  UpperLimit=n  LowerLimit=0
  Sum1 : Sum  Inputs=1  InputSameDT=on  SaturateOnIntegerOverflow=on  OutDataTypeStr=Inherit: Same as first input
  Sum2 : Sum  Inputs=+-  InputSameDT=on  SaturateOnIntegerOverflow=on  OutDataTypeStr=Inherit: Same as first input
  Unit Delay1 : UnitDelay  SampleTime=Ts  HasFrameUpgradeWarning=on
  Unit Delay3 : UnitDelay  InitialCondition=Vc_Initial  SampleTime=Ts  HasFrameUpgradeWarning=on
  Unit Delay4 : UnitDelay  InitialCondition=Vc_Initial  SampleTime=Ts  HasFrameUpgradeWarning=on
  Vp : spsControlledVoltageSourceLib/Controlled Voltage Source  Initialize=off  Source_Type=AC  Amplitude=0  Phase=0  Frequency=0  Measurements=None
  Vp1 : spsControlledVoltageSourceLib/Controlled Voltage Source  Initialize=off  Source_Type=AC  Amplitude=0  Phase=0  Frequency=0  Measurements=None
  1 : PMIOPort  Side=Left
  2 : PMIOPort  Port=2  Side=Left
  Vc : Outport  VectorParamsAs1DForOutWhenUnconnected=off
  wires:
  N/1 -> Saturation1/1
  [Imod] -> Mux/1
  Unit Delay3/1 -> Sum2/2
  Unit Delay4/1 -> Unit Delay3/1, Gain2/1
  Gain2/1 -> Sum2/1
  Gain/1 -> Discrete-Time Integrator/1
  Discrete-Time Integrator/1 -> Unit Delay4/1
  Mux/1 -> Unit Delay1/1
  Product2/1 -> Demux/1
  Demux/1 -> [Vin]
  Demux/2 -> [Vbl]
  [Vin] -> Vp/1
  Current Measurement1/1 -> [Imod]
  Current Measurement2/1 -> [Icap]
  [Vbl] -> Vp1/1
  [Icap] -> Mux/2
  Unit Delay1/1 -> Product1/2
  Saturation1/1 -> Product1/1, Product2/1
  Product1/1 -> Sum1/1
  Sum2/1 -> Product2/2, Vc/1
  Sum1/1 -> Gain/1
  connections:
  1/RConn1 -- Vp/RConn1
  Vp/LConn1 -- Current Measurement1/LConn1
  Current Measurement1/RConn1 -- Dp/LConn1 -- Dp2/RConn1
  Current Measurement2/LConn1 -- Dp/RConn1
  Vp1/RConn1 -- Current Measurement2/RConn1
  Vp1/LConn1 -- 2/RConn1 -- Dp2/LConn1

== system lib_dGrid/MMC-configurable control modes/Half-Bridge MMC Cp/HalfBridgeMMC_Agt_Discrete ==
  N : Inport  PortDimensions=2
  Current Measurement1 : spsCurrentMeasurementLib/Current Measurement  PhasorSimulation=off  OutputType=Complex  PSBequivalent=0
  Current Measurement2 : spsCurrentMeasurementLib/Current Measurement  PhasorSimulation=off  OutputType=Complex  PSBequivalent=0
  Demux : Demux  Outputs=2
  Discrete-Time Integrator : DiscreteIntegrator  IntegratorMethod=Integration: Trapezoidal  gainval=1  InitialCondition=Vc_Initial  SampleTime=Ts  UpperSaturationLimit=5000  LowerSaturationLimit=500  ICPrevOutput=DiscIntNeverNeededParam  ICPrevScaledInput=DiscIntNeverNeededParam
  Dp : spsDiodeLib/Diode  Ron=Ron_Diode  Lon=0  Vf=Vf_Diode  IC=0  UseSnubber=off  Rs=Rs_Diode  Cs=Cs_Diode  Measurements=off
  Dp2 : spsDiodeLib/Diode  Ron=Ron_Diode  Lon=0  Vf=Vf_Diode  IC=0  UseSnubber=off  Rs=Rs_Diode  Cs=Cs_Diode  Measurements=off
  Gain : Gain  Gain=1/(C*n)
  Gain2 : Gain  Gain=2
  Mux : Mux  Inputs=2
  Product1 : Product
  Product2 : Product
  Saturation1 : Saturate  UpperLimit=n  LowerLimit=0
  Sum1 : Sum  Inputs=1  InputSameDT=on  SaturateOnIntegerOverflow=on  OutDataTypeStr=Inherit: Same as first input
  Sum2 : Sum  Inputs=+-  InputSameDT=on  SaturateOnIntegerOverflow=on  OutDataTypeStr=Inherit: Same as first input
  Unit Delay1 : UnitDelay  SampleTime=Ts  HasFrameUpgradeWarning=on
  Unit Delay3 : UnitDelay  InitialCondition=Vc_Initial  SampleTime=Ts  HasFrameUpgradeWarning=on
  Unit Delay4 : UnitDelay  InitialCondition=Vc_Initial  SampleTime=Ts  HasFrameUpgradeWarning=on
  Vp : spsControlledVoltageSourceLib/Controlled Voltage Source  Initialize=off  Source_Type=AC  Amplitude=0  Phase=0  Frequency=0  Measurements=None
  Vp1 : spsControlledVoltageSourceLib/Controlled Voltage Source  Initialize=off  Source_Type=AC  Amplitude=0  Phase=0  Frequency=0  Measurements=None
  1 : PMIOPort  Side=Left
  2 : PMIOPort  Port=2  Side=Left
  Vc : Outport  VectorParamsAs1DForOutWhenUnconnected=off
  wires:
  Sum1/1 -> Gain/1
  Sum2/1 -> Vc/1, Product2/2
  Product1/1 -> Sum1/1
  Saturation1/1 -> Product2/1, Product1/1
  Unit Delay1/1 -> Product1/2
  [Icap] -> Mux/2
  [Vbl] -> Vp1/1
  Current Measurement2/1 -> [Icap]
  Current Measurement1/1 -> [Imod]
  [Vin] -> Vp/1
  Demux/2 -> [Vbl]
  Demux/1 -> [Vin]
  Product2/1 -> Demux/1
  Mux/1 -> Unit Delay1/1
  Discrete-Time Integrator/1 -> Unit Delay4/1
  Gain/1 -> Discrete-Time Integrator/1
  Gain2/1 -> Sum2/1
  Unit Delay4/1 -> Gain2/1, Unit Delay3/1
  Unit Delay3/1 -> Sum2/2
  [Imod] -> Mux/1
  N/1 -> Saturation1/1
  connections:
  Dp2/LConn1 -- 2/RConn1 -- Vp1/LConn1
  Vp1/RConn1 -- Current Measurement2/RConn1
  Current Measurement2/LConn1 -- Dp/RConn1
  Dp2/RConn1 -- Dp/LConn1 -- Current Measurement1/RConn1
  Vp/LConn1 -- Current Measurement1/LConn1
  1/RConn1 -- Vp/RConn1
